simulink model "Quasi_Static_approach_powertrain"  (R2021a)
settings: Solver=VariableStepAuto  StartTime=0.0  StopTime=1200  MaxStep=0.01  RelTol=1e-3
values from neighbouring files (symbols this model uses):
  Area_V = 3.8056    [Powertrain.m]
  B_Voltage = 364    [Powertrain.m]
  Cd = 0.28    [Powertrain.m]
  cell_capacity = 33.1    [Powertrain.m]
  cell_vol = 3.8    [Powertrain.m]
  Crr = 0.015    [Powertrain.m]
  D_mass = 80    [Powertrain.m]
  G_R = 7.8    [Powertrain.m]
  Mass_V = 1710.655    [Powertrain.m]
  Motor_cont_efficiency = Motor_Cont(1:15,2:16)    [Powertrain.m]
  Motor_cont_efficiency_regen = Motor_Cont_regen(1:15,2:16)    [Powertrain.m]
  Motor_cont_speed = Motor_Cont(1:15,1)    [Powertrain.m]
  Motor_cont_speed_regen = Motor_Cont_regen(1:15,1)    [Powertrain.m]
  Motor_cont_torque = Motor_Cont(1:15,17)    [Powertrain.m]
  Motor_cont_torque_regen = Motor_Cont_regen(1:15,17)    [Powertrain.m]
  Motor_efficiency = Motor_eff(1:15,2:16)    [Powertrain.m]
  Motor_efficiency_regen = Motor_eff_regen(1:15,2:16)    [Powertrain.m]
  Motor_speed = Motor_eff(1:15,1)    [Powertrain.m]
  Motor_speed_regen = Motor_eff_regen(1:15,1)    [Powertrain.m]
  Motor_torque = Motor_eff(1:15,17)    [Powertrain.m]
  Motor_torque_regen = Motor_eff_regen(1:15,17)    [Powertrain.m]
  Rho = 1.225    [Powertrain.m]
  Rw = 0.2032    [Powertrain.m]
  T_eff = 0.85    [Powertrain.m]
settings Model: Creator=LENOVO  LastModifiedBy=LENOVO

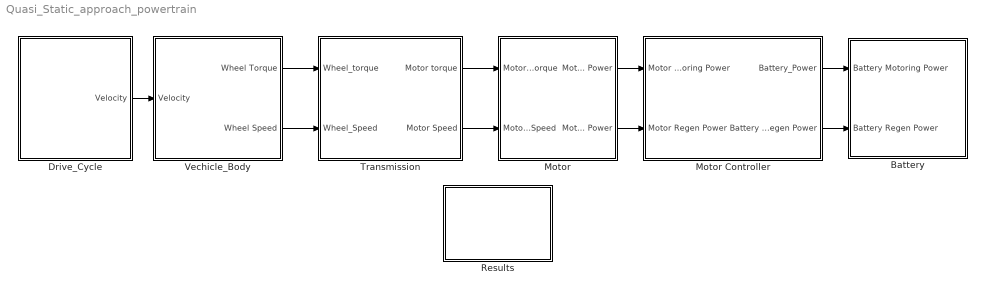
== system Quasi_Static_approach_powertrain ==
  Battery : Subsystem
  Drive_Cycle : Subsystem
  Motor : Subsystem
  Motor Controller : Subsystem
  Results : Subsystem
  Transmission : Subsystem
  Vechicle_Body : Subsystem
  wires:
  Drive_Cycle/1("Velocity ") -> Vechicle_Body/1("Velocity ")
  Vechicle_Body/1(Wheel Torque) -> Transmission/1(Wheel_torque)
  Vechicle_Body/2(Wheel Speed) -> Transmission/2(Wheel_Speed)
  Transmission/1(Motor torque) -> Motor/1(Motor Torque)
  Transmission/2(Motor Speed) -> Motor/2(Motor Speed)
  Motor/1(Motor Power) -> Motor Controller/1(Motor Motoring Power)
  Motor Controller/1(Battery_Power) -> Battery/1(Battery Motoring Power)
  Motor/2(Motor Regen Power) -> Motor Controller/2(Motor Regen Power)
  Motor Controller/2(Battery Regen Power) -> Battery/2(Battery Regen Power)

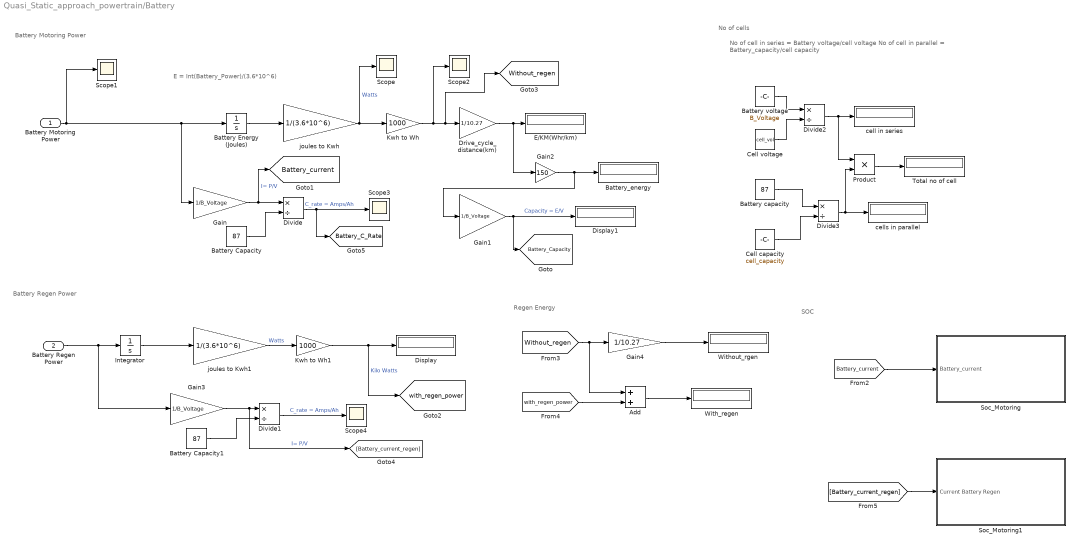
== system Quasi_Static_approach_powertrain/Battery ==
  note: No of cells
  note: No of cell in series = Battery voltage/cell voltage
      | No of cell in parallel = Battery_capacity/cell capacity
  note: SOC
  note: Regen Energy
  note: Battery Regen Power
  note: Battery Motoring Power
  note: E = Int(Battery_Power)/(3.6*10^6)
  Battery Motoring Power : Inport
  Battery Regen Power : Inport  Port=2
  Add : Sum
  Battery Capacity : Constant  Value=87
  Battery Capacity1 : Constant  Value=87
  Battery Energy (Joules) : Integrator
  Battery capacity : Constant  Value=87
  Battery voltage : Constant  Value=B_Voltage
  Battery_energy : Display
  Cell capacity : Constant  Value=cell_capacity
  Cell voltage : Constant  Value=cell_vol
  Display : Display
  Display1 : Display
  Divide{,1..3} (4 alike) : Product  Inputs=*/
  Drive_cycle_distance(km) : Gain  Gain=1/10.27
  E/KM(Whr/km) : Display
  Gain : Gain  Gain=1/B_Voltage
  Gain1 : Gain  Gain=1/B_Voltage
  Gain2 : Gain  Gain=150
  Gain3 : Gain  Gain=1/B_Voltage
  Gain4 : Gain  Gain=1/10.27
  Integrator : Integrator
  Kwh to Wh : Gain  Gain=1000
  Kwh to Wh1 : Gain  Gain=1000
  Product : Product
  Scope{,1..4} (5 alike) : Scope
  Soc_Motoring : Subsystem
  Soc_Motoring1 : Subsystem
  Total no of cell : Display
  With_regen : Display
  Without_rgen : Display
  cell in series : Display
  cells in parallel : Display
  joules to Kwh : Gain  Gain=1/(3.6*10^6)
  joules to Kwh1 : Gain  Gain=1/(3.6*10^6)
  tag scope: Battery_C_Rate=global, Battery_Capacity=global, Battery_current=global, Without_regen=global, with_regen_power=global
  wires:
  Battery Motoring Power/1 -> Gain/1, Battery Energy (Joules)/1, Scope1/1
  Battery Energy (Joules)/1 -> joules to Kwh/1
  joules to Kwh/1 -> Scope/1, Kwh to Wh/1  "Watts"
  Kwh to Wh/1 -> Scope2/1, [Without_regen], Drive_cycle_distance(km)/1
  Drive_cycle_distance(km)/1 -> Gain2/1, E/KM(Whr/km)/1
  Gain2/1 -> Gain1/1, Battery_energy/1
  Battery Regen Power/1 -> Gain3/1, Integrator/1
  Integrator/1 -> joules to Kwh1/1
  joules to Kwh1/1 -> Kwh to Wh1/1  "Watts"
  Kwh to Wh1/1 -> [with_regen_power], Display/1  "Kilo Watts"
  Gain/1 -> Divide/1, [Battery_current]  "I= P/V"
  Gain1/1 -> [Battery_Capacity], Display1/1  "Capacity = E/V"
  Battery Capacity/1 -> Divide/2
  Divide/1 -> Scope3/1, [Battery_C_Rate]  "C_rate = Amps/Ah"
  Divide1/1 -> Scope4/1  "C_rate = Amps/Ah"
  Gain3/1 -> [Battery_current_regen], Divide1/1  "I= P/V"
  Battery Capacity1/1 -> Divide1/2
  [Battery_current] -> Soc_Motoring/1(Battery_current)
  [Without_regen] -> Add/1, Gain4/1
  [with_regen_power] -> Add/2
  Gain4/1 -> Without_rgen/1
  Add/1 -> With_regen/1
  Battery voltage/1 -> Divide2/1
  Cell voltage/1 -> Divide2/2
  Divide2/1 -> Product/1, cell in series/1
  Battery capacity/1 -> Divide3/1
  Cell capacity/1 -> Divide3/2
  Divide3/1 -> Product/2, cells in parallel/1
  Product/1 -> Total no of cell/1
  [Battery_current_regen] -> Soc_Motoring1/1(Current Battery Regen)

== system Quasi_Static_approach_powertrain/Drive_Cycle ==
  Artemis_Rural_Drive_Cycle : FromWorkspace  VariableName=data2
  Artemis_Urban_Drive_Cycle : FromWorkspace  VariableName=data1
  Constant : Constant
  Drive Cycle : FromWorkspace  VariableName=data
  Multiport Switch : MultiPortSwitch
  "Velocity " : Outport
  wires:
  Constant/1 -> Multiport Switch/1
  Drive Cycle/1 -> Multiport Switch/2
  Artemis_Urban_Drive_Cycle/1 -> Multiport Switch/3
  Artemis_Rural_Drive_Cycle/1 -> Multiport Switch/4
  Multiport Switch/1 -> "Velocity "/1

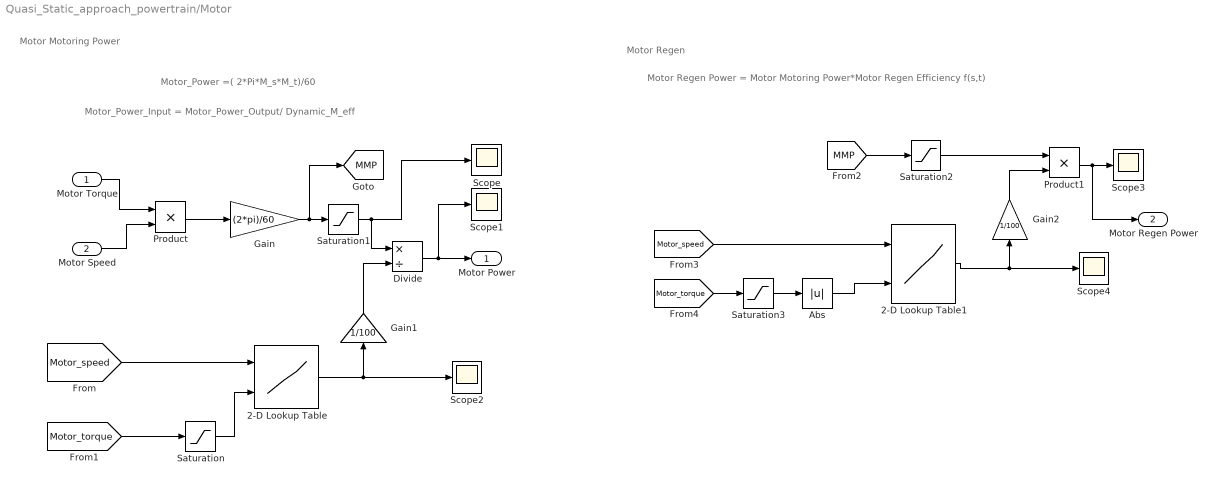
== system Quasi_Static_approach_powertrain/Motor ==
  note: Motor Regen
  note: Motor Regen Power = Motor Motoring Power*Motor Regen Efficiency f(s,t)
  note: Motor Motoring Power
  note: Motor_Power_Input = Motor_Power_Output/ Dynamic_M_eff
  note: Motor_Power =( 2*Pi*M_s*M_t)/60
  Motor Torque : Inport
  Motor Speed : Inport  Port=2
  2-D Lookup Table : Lookup_n-D  BreakpointsForDimension1=Motor_speed  BreakpointsForDimension2=Motor_torque  Table=Motor_efficiency  InternalRulePriority=Speed  RndMeth=Simplest  InputSameDT=on
      settings: InputPortMap=u0,u1
  2-D Lookup Table1 : Lookup_n-D  BreakpointsForDimension1=Motor_speed_regen  BreakpointsForDimension2=Motor_torque_regen  Table=Motor_efficiency_regen  InternalRulePriority=Speed  RndMeth=Simplest  InputSameDT=on
      settings: InputPortMap=u0,u1
  Abs : Abs
  Divide : Product  Inputs=*/
  Gain : Gain  Gain=(2*pi)/60
  Gain1 : Gain  Gain=1/100
  Gain2 : Gain  Gain=1/100
  Product : Product
  Product1 : Product
  Saturation : Saturate  UpperLimit=inf  LowerLimit=0
  Saturation1 : Saturate  UpperLimit=inf  LowerLimit=0
  Saturation2 : Saturate  UpperLimit=0  LowerLimit=-inf
  Saturation3 : Saturate  UpperLimit=0  LowerLimit=-inf
  Scope{,1..4} (5 alike) : Scope
  Motor Power : Outport
  Motor Regen Power : Outport  Port=2
  tag scope: MMP=global
  wires:
  Motor Torque/1 -> Product/1
  Motor Speed/1 -> Product/2
  Product/1 -> Gain/1
  Divide/1 -> Scope1/1, Motor Power/1
  [Motor_torque] -> Saturation/1
  [Motor_speed] -> 2-D Lookup Table/1
  Saturation/1 -> 2-D Lookup Table/2
  2-D Lookup Table/1 -> Gain1/1, Scope2/1
  Gain1/1 -> Divide/2
  Gain/1 -> [MMP], Saturation1/1
  Saturation1/1 -> Scope/1, Divide/1
  [MMP] -> Saturation2/1
  [Motor_speed] -> 2-D Lookup Table1/1
  [Motor_torque] -> Saturation3/1
  Saturation3/1 -> Abs/1
  Abs/1 -> 2-D Lookup Table1/2
  2-D Lookup Table1/1 -> Scope4/1, Gain2/1
  Saturation2/1 -> Product1/1
  Gain2/1 -> Product1/2
  Product1/1 -> Motor Regen Power/1, Scope3/1

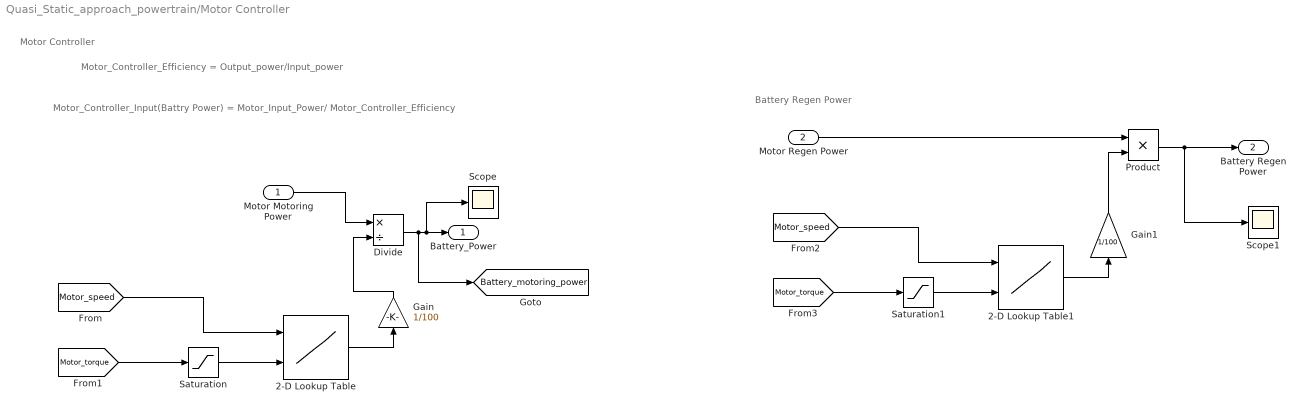
== system Quasi_Static_approach_powertrain/Motor Controller ==
  note: Battery Regen Power
  note: Motor Controller
  note: Motor_Controller_Input(Battry Power) = Motor_Input_Power/ Motor_Controller_Efficiency
  note: Motor_Controller_Efficiency = Output_power/Input_power
  Motor Motoring Power : Inport
  Motor Regen Power : Inport  Port=2
  2-D Lookup Table : Lookup_n-D  BreakpointsForDimension1=Motor_cont_speed  BreakpointsForDimension2=Motor_cont_torque  Table=Motor_cont_efficiency  InternalRulePriority=Speed  RndMeth=Simplest  InputSameDT=on
      settings: InputPortMap=u0,u1
  2-D Lookup Table1 : Lookup_n-D  BreakpointsForDimension1=Motor_cont_speed_regen  BreakpointsForDimension2=Motor_cont_torque_regen  Table=Motor_cont_efficiency_regen  InternalRulePriority=Speed  RndMeth=Simplest  InputSameDT=on
      settings: InputPortMap=u0,u1
  Divide : Product  Inputs=*/
  Gain : Gain  Gain=1/100
  Gain1 : Gain  Gain=1/100
  Product : Product
  Saturation : Saturate  UpperLimit=inf  LowerLimit=0
  Saturation1 : Saturate  UpperLimit=inf  LowerLimit=0
  Scope : Scope
  Scope1 : Scope
  Battery_Power : Outport
  Battery Regen Power : Outport  Port=2
  tag scope: Battery_motoring_power=global
  wires:
  Motor Motoring Power/1 -> Divide/1
  Gain/1 -> Divide/2
  Divide/1 -> Battery_Power/1, Scope/1, [Battery_motoring_power]
  [Motor_torque] -> Saturation/1
  Saturation/1 -> 2-D Lookup Table/2
  [Motor_speed] -> 2-D Lookup Table/1
  2-D Lookup Table/1 -> Gain/1
  [Motor_torque] -> Saturation1/1
  [Motor_speed] -> 2-D Lookup Table1/1
  Saturation1/1 -> 2-D Lookup Table1/2
  2-D Lookup Table1/1 -> Gain1/1
  Gain1/1 -> Product/2
  Motor Regen Power/1 -> Product/1
  Product/1 -> Battery Regen Power/1, Scope1/1

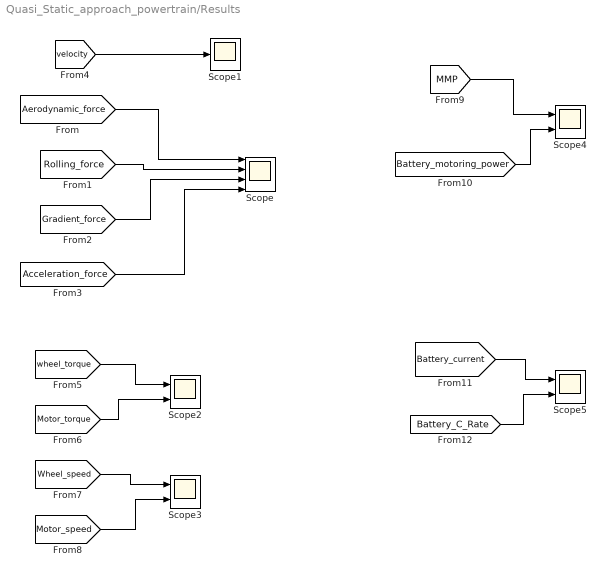
== system Quasi_Static_approach_powertrain/Results ==
  Scope : Scope  NumInputPorts=4
  Scope1 : Scope
  Scope{2..5} (4 alike) : Scope  NumInputPorts=2
  wires:
  [Aerodynamic_force] -> Scope/1
  [Rolling_force] -> Scope/2
  [Gradient_force] -> Scope/3
  [Acceleration_force] -> Scope/4
  [velocity] -> Scope1/1
  [wheel_torque] -> Scope2/1
  [Motor_torque] -> Scope2/2
  [Wheel_speed] -> Scope3/1
  [Motor_speed] -> Scope3/2
  [MMP] -> Scope4/1
  [Battery_motoring_power] -> Scope4/2
  [Battery_current] -> Scope5/1
  [Battery_C_Rate] -> Scope5/2

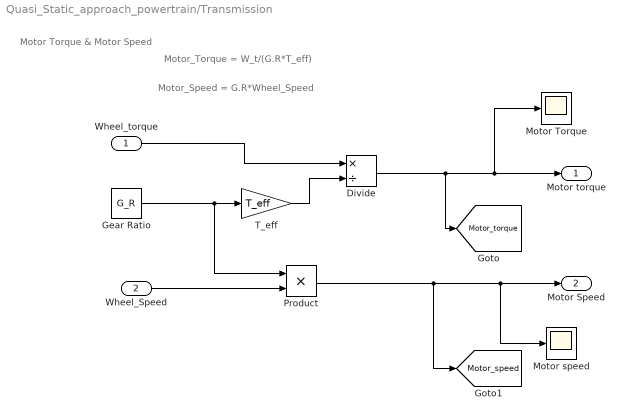
== system Quasi_Static_approach_powertrain/Transmission ==
  note: Motor Torque & Motor Speed
  note: Motor_Speed = G.R*Wheel_Speed
  note: Motor_Torque = W_t/(G.R*T_eff)
  Wheel_torque : Inport
  Wheel_Speed : Inport  Port=2
  Divide : Product  Inputs=*/
  Gear Ratio : Constant  Value=G_R
  Motor Torque : Scope
  Motor speed : Scope
  Product : Product
  T_eff : Gain  Gain=T_eff
  Motor torque : Outport
  Motor Speed : Outport  Port=2
  tag scope: Motor_speed=global, Motor_torque=global
  wires:
  Gear Ratio/1 -> Product/1, T_eff/1
  Wheel_torque/1 -> Divide/1
  T_eff/1 -> Divide/2
  Divide/1 -> [Motor_torque], Motor Torque/1, Motor torque/1
  Wheel_Speed/1 -> Product/2
  Product/1 -> [Motor_speed], Motor speed/1, Motor Speed/1

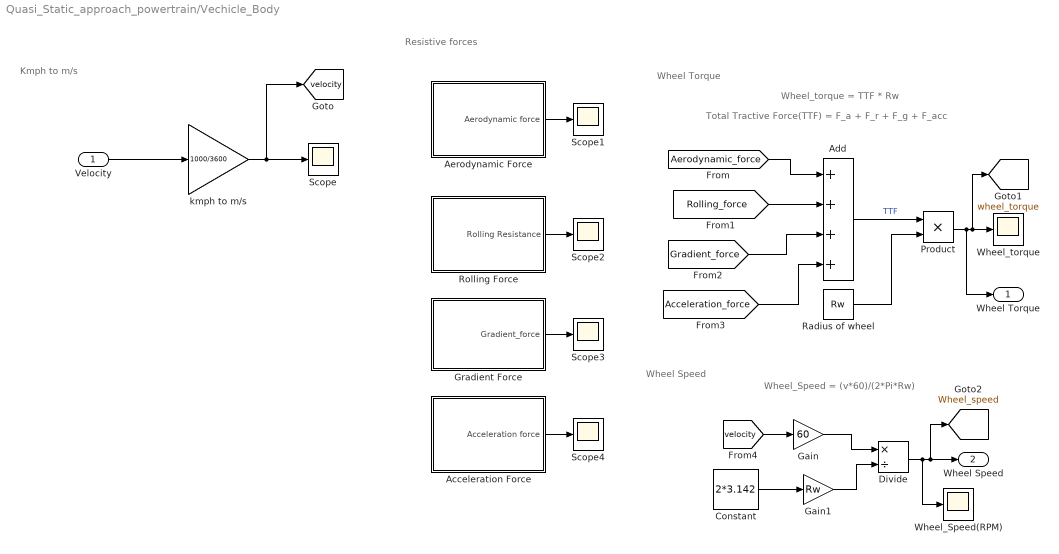
== system Quasi_Static_approach_powertrain/Vechicle_Body ==
  note: Wheel Speed
  note: Wheel_Speed = (v*60)/(2*Pi*Rw)
  note: Wheel Torque
  note: Resistive forces
  note: Wheel_torque = TTF * Rw
  note: Total Tractive Force(TTF) = F_a + F_r + F_g + F_acc
  note: Kmph to m/s
  "Velocity " : Inport
  Acceleration Force : Subsystem
  Add : Sum  Inputs=++++
  Aerodynamic Force : Subsystem
  Constant : Constant  Value=2*3.142
  Divide : Product  Inputs=*/
  Gain : Gain  Gain=60
  Gain1 : Gain  Gain=Rw
  Gradient Force : Subsystem
  Product : Product
  Radius of wheel : Constant  Value=Rw
  Rolling Force : Subsystem
  Scope{,1..4} (5 alike) : Scope
  Wheel_Speed(RPM) : Scope
  Wheel_torque : Scope
  kmph to m/s : Gain  Gain=1000/3600
  Wheel Torque : Outport
  Wheel Speed : Outport  Port=2
  tag scope: Wheel_speed=global, velocity=global, wheel_torque=global
  wires:
  "Velocity "/1 -> kmph to m/s/1
  kmph to m/s/1 -> [velocity], Scope/1
  Gradient Force/1(Gradient_force) -> Scope3/1
  Acceleration Force/1(Acceleration force) -> Scope4/1
  [Aerodynamic_force] -> Add/1
  [Rolling_force] -> Add/2
  [Gradient_force] -> Add/3
  [Acceleration_force] -> Add/4
  Add/1 -> Product/1  "TTF"
  Radius of wheel/1 -> Product/2
  Product/1 -> Wheel Torque/1, [wheel_torque], Wheel_torque/1
  [velocity] -> Gain/1
  Constant/1 -> Gain1/1
  Gain/1 -> Divide/1
  Gain1/1 -> Divide/2
  Divide/1 -> Wheel_Speed(RPM)/1, [Wheel_speed], Wheel Speed/1
  Aerodynamic Force/1(Aerodynamic force) -> Scope1/1
  Rolling Force/1(Rolling Resistance) -> Scope2/1

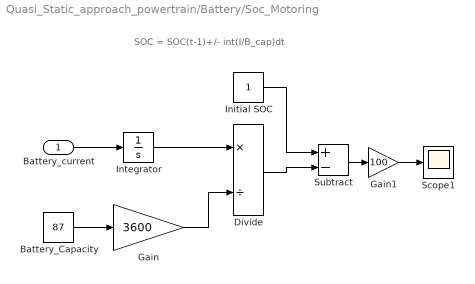
== system Quasi_Static_approach_powertrain/Battery/Soc_Motoring ==
  note: SOC = SOC(t-1)+/- int(I/B_cap)dt
  Battery_current : Inport
  Battery_Capacity : Constant  Value=87
  Divide : Product  Inputs=*/
  Gain : Gain  Gain=3600
  Gain1 : Gain  Gain=100
  Initial SOC : Constant
  Integrator : Integrator
  Scope1 : Scope
  Subtract : Sum  Inputs=+-
  wires:
  Initial SOC/1 -> Subtract/1
  Battery_current/1 -> Integrator/1
  Battery_Capacity/1 -> Gain/1
  Integrator/1 -> Divide/1
  Gain/1 -> Divide/2
  Divide/1 -> Subtract/2
  Subtract/1 -> Gain1/1
  Gain1/1 -> Scope1/1

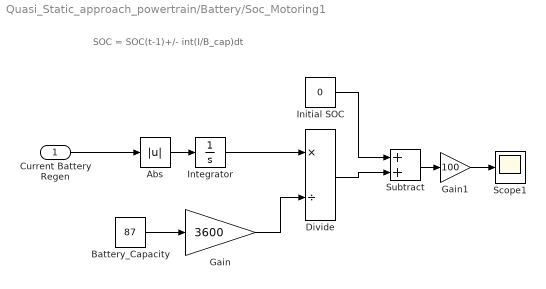
== system Quasi_Static_approach_powertrain/Battery/Soc_Motoring1 ==
  note: SOC = SOC(t-1)+/- int(I/B_cap)dt
  Current Battery Regen : Inport
  Abs : Abs
  Battery_Capacity : Constant  Value=87
  Divide : Product  Inputs=*/
  Gain : Gain  Gain=3600
  Gain1 : Gain  Gain=100
  Initial SOC : Constant  Value=0
  Integrator : Integrator  InitialCondition=1
  Scope1 : Scope
  Subtract : Sum
  wires:
  Divide/1 -> Subtract/2
  Battery_Capacity/1 -> Gain/1
  Gain/1 -> Divide/2
  Gain1/1 -> Scope1/1
  Initial SOC/1 -> Subtract/1
  Subtract/1 -> Gain1/1
  Integrator/1 -> Divide/1
  Current Battery Regen/1 -> Abs/1
  Abs/1 -> Integrator/1

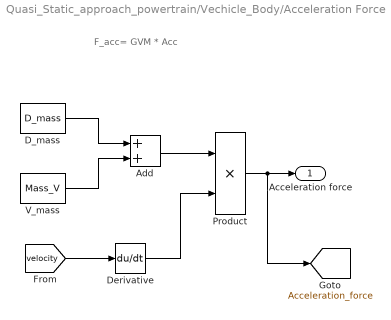
== system Quasi_Static_approach_powertrain/Vechicle_Body/Acceleration Force ==
  note: F_acc= GVM * Acc
  Add : Sum
  D_mass : Constant  Value=D_mass
  Derivative : Derivative
  Product : Product
  V_mass : Constant  Value=Mass_V
  Acceleration force : Outport
  tag scope: Acceleration_force=global
  wires:
  D_mass/1 -> Add/1
  V_mass/1 -> Add/2
  [velocity] -> Derivative/1
  Add/1 -> Product/1
  Derivative/1 -> Product/2
  Product/1 -> [Acceleration_force], Acceleration force/1

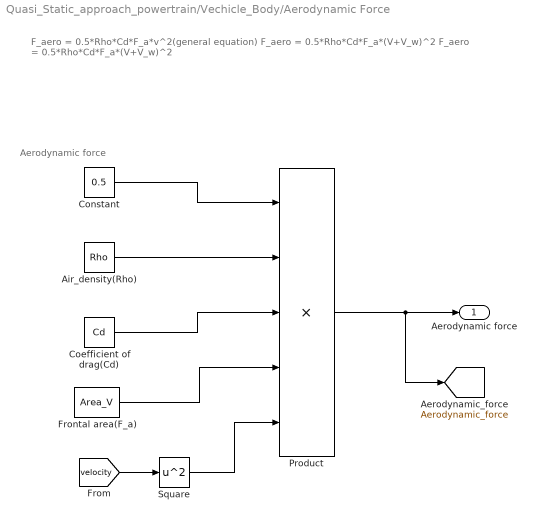
== system Quasi_Static_approach_powertrain/Vechicle_Body/Aerodynamic Force ==
  note: Aerodynamic force
  note: F_aero = 0.5*Rho*Cd*F_a*v^2(general equation)
      | F_aero = 0.5*Rho*Cd*F_a*(V+V_w)^2
      | F_aero = 0.5*Rho*Cd*F_a*(V+V_w)^2
  Air_density(Rho) : Constant  Value=Rho
  Coefficient of drag(Cd) : Constant  Value=Cd
  Constant : Constant  Value=0.5
  Frontal area(F_a) : Constant  Value=Area_V
  Product : Product  Inputs=5
  Square : Math  Operator=square  SaturateOnIntegerOverflow=on
  Aerodynamic force : Outport
  tag scope: Aerodynamic_force=global
  wires:
  [velocity] -> Square/1
  Constant/1 -> Product/1
  Air_density(Rho)/1 -> Product/2
  Coefficient of drag(Cd)/1 -> Product/3
  Frontal area(F_a)/1 -> Product/4
  Square/1 -> Product/5
  Product/1 -> [Aerodynamic_force], Aerodynamic force/1

== system Quasi_Static_approach_powertrain/Vechicle_Body/Gradient Force ==
  note: Gradient_force = GVW*Sin(Theta)
  Constant : Constant  Value=0
  Product : Product
  Sin : Trigonometry
  Gradient_force : Outport
  tag scope: Gradient_force=global
  wires:
  Constant/1 -> Sin/1
  [GVW] -> Product/1
  Sin/1 -> Product/2
  Product/1 -> [Gradient_force], Gradient_force/1

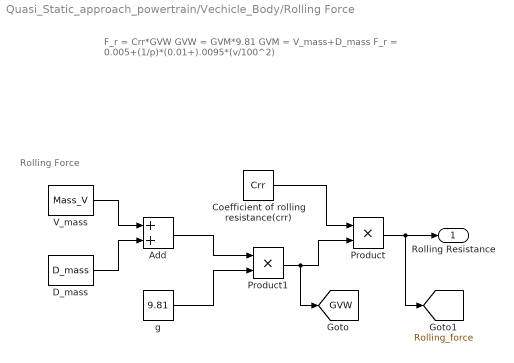
== system Quasi_Static_approach_powertrain/Vechicle_Body/Rolling Force ==
  note: Rolling Force
  note: F_r = Crr*GVW
      | GVW = GVM*9.81
      | GVM = V_mass+D_mass
      | F_r = 0.005+(1/p)*(0.01+).0095*(v/100^2)
  Add : Sum
  Coefficient of rolling resistance(crr) : Constant  Value=Crr
  D_mass : Constant  Value=D_mass
  Product : Product
  Product1 : Product
  V_mass : Constant  Value=Mass_V
  g : Constant  Value=9.81
  Rolling Resistance : Outport
  tag scope: GVW=global, Rolling_force=global
  wires:
  V_mass/1 -> Add/1
  D_mass/1 -> Add/2
  Add/1 -> Product1/1
  g/1 -> Product1/2
  Coefficient of rolling resistance(crr)/1 -> Product/1
  Product1/1 -> [GVW], Product/2
  Product/1 -> [Rolling_force], Rolling Resistance/1
